simulink model "PIdf"  (R2016a)
settings: Solver=FixedStepDiscrete  StartTime=0.0  StopTime=20
undefined symbols (not defined in the file or in its folder): DiscIntNeverNeededParam
libraries: simulink x1, fuzblock x1
settings Model: Creator=PC  LastModifiedBy=PC
settings SolverCC: MaxConsecutiveZCs=10000  SolverJacobianMethodControl=FullAnalytical  ZeroCrossControl=DisableAll  ZeroCrossAlgorithm=Adaptive  AutoInsertRateTranBlk=on
settings DataIOCC: LimitDataPoints=on  SaveOutput=off  SaveTime=off  Refine=10
settings OptimizationCC: ExpressionDepthLimit=2147483647  LifeSpan=1
settings DebuggingCC: UnderspecifiedInitializationDetection=Classic  MergeDetectMultiDrivingBlocksExec=none  FcnCallInpInsideContextMsg=EnableAllAsWarning  AllowSymbolicDim=off  StateNameClashWarn=warning
settings GRTTargetCC: CombineOutputUpdateFcns=off  GRTInterface=on

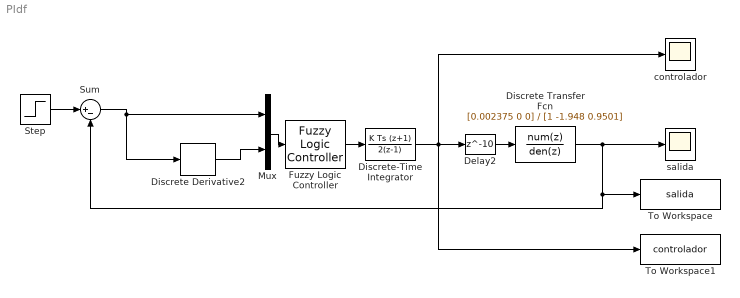
== system PIdf ==
  Delay2 : Delay  DelayLength=10  SampleTime=0.05
  Discrete Transfer Fcn : DiscreteTransferFcn  Numerator=[0.002375 0 0]  Denominator=[1 -1.948 0.9501]  SampleTime=0.05
  Discrete Derivative2 : simulink/Discrete/Discrete Derivative  gainval=1.0  ICPrevScaledInput=0.0  OutMin=[]  OutMax=[]  OutDataType=fixdt(1, 16)  OutScaling=2^-10  DoSatur=off
  Discrete-Time Integrator : DiscreteIntegrator  IntegratorMethod=Integration: Trapezoidal  InitialConditionSetting=State (most efficient)  SampleTime=0.05  ICPrevOutput=DiscIntNeverNeededParam  ICPrevScaledInput=DiscIntNeverNeededParam
  Fuzzy Logic Controller : fuzblock/Fuzzy Logic  Controller  fis='PI.fis'
  Mux : Mux  Inputs=2
  Step : Step  Time=0  SampleTime=0
  Sum : Sum  Inputs=|+-
  To Workspace : ToWorkspace  VariableName=salida  SaveFormat=Timeseries  SampleTime=-1
  To Workspace1 : ToWorkspace  VariableName=controlador  SaveFormat=Timeseries  SampleTime=-1
  controlador : Scope
  "salida " : Scope
  wires:
  Discrete Transfer Fcn/1 -> "salida "/1, Sum/2, To Workspace/1
  Fuzzy Logic Controller/1 -> Discrete-Time Integrator/1
  Mux/1 -> Fuzzy Logic Controller/1
  Discrete-Time Integrator/1 -> controlador/1, Delay2/1, To Workspace1/1
  Sum/1 -> Discrete Derivative2/1, Mux/1
  Discrete Derivative2/1 -> Mux/2
  Delay2/1 -> Discrete Transfer Fcn/1
  Step/1 -> Sum/1
